simulink model "ACC_mod"  (R2025b)
settings: Solver=FixedStepAuto  StartTime=0  StopTime=SVT_StopTime  FixedStep=0.01  RelTol=1e-3
undefined symbols (not defined in the file): SVT_StepTime
settings Model: DataDictionary=ACC.sldd  Creator=spadhi  LastModifiedBy=spadhi
settings DataIOCC: TimeSaveName=SVT_tout  SignalLoggingName=SVT_logsout  DSMLoggingName=SVT_dsmout
settings DebuggingCC: SignalRangeChecking=warning  ModelReferenceIOMismatchMessage=error
settings ModelReferenceCC: UpdateModelReferenceTargets=IfOutOfDate  ModelReferenceNumInstancesAllowed=Single
settings ConfigComp: CovEnable=on  CovScope=ReferencedModels  CovIncludeTopModel=off  CovMetricSettings=dcmwe  CovHTMLOptions=-sRT=0 -sVT=0 -aTS=1 -bRG=1 -bTC=1 -hTR=0 -nFC=0 -scm=1 -bcm=1 -xEv=0  CovCumulativeReport=on  CovModelRefEnable=all

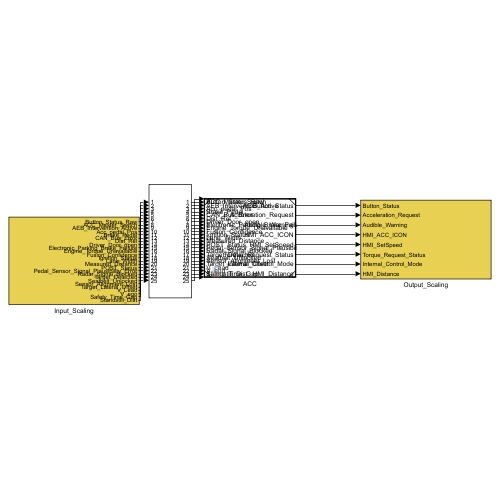
[thumbnail: Simulink's stored preview of the top-level diagram]
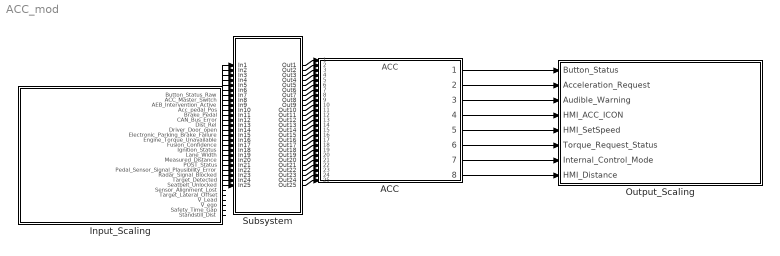
== system ACC_mod ==
  ACC : ModelReference  ModelNameDialog=ACC.slx  SimulationMode=Normal  ModelReferenceVersion=1.273
  Input_Scaling : Subsystem
  Output_Scaling : Subsystem
  Subsystem : Subsystem
  wires:
  Input_Scaling/1(Button_Status_Raw) -> Subsystem/1(In1)
  Input_Scaling/2(ACC_Master_Switch) -> Subsystem/2(In2)
  Input_Scaling/3(AEB_Intervention_Active) -> Subsystem/3(In3)
  Input_Scaling/4(Acc_pedal_Pos) -> Subsystem/4(In4)
  Input_Scaling/5(Brake_Pedal) -> Subsystem/5(In5)
  Input_Scaling/6(CAN_Bus_Error) -> Subsystem/6(In6)
  Input_Scaling/7(Dist_Rel) -> Subsystem/7(In7)
  Input_Scaling/8(Driver_Door_open) -> Subsystem/8(In8)
  Input_Scaling/9(Electronic_Parking_Brake_Failure) -> Subsystem/9(In9)
  Input_Scaling/10(Engine_Torque_Unavailable) -> Subsystem/10(In10)
  Input_Scaling/11(Fusion_Confidence) -> Subsystem/11(In11)
  Input_Scaling/12(Ignition_Status) -> Subsystem/12(In12)
  Input_Scaling/13(Lane_Width) -> Subsystem/13(In13)
  Input_Scaling/14(Measured_Distance) -> Subsystem/14(In14)
  Input_Scaling/15(POST_Status) -> Subsystem/15(In15)
  Input_Scaling/16(Pedal_Sensor_Signal_Plausibility_Error) -> Subsystem/16(In16)
  Input_Scaling/17(Radar_Signal_Blocked) -> Subsystem/17(In17)
  Input_Scaling/18(Target_Detected) -> Subsystem/18(In18)
  Input_Scaling/19(Seatbelt_Unlocked) -> Subsystem/19(In19)
  Input_Scaling/20(Sensor_Alignment_Lost) -> Subsystem/20(In20)
  Input_Scaling/21(Target_Lateral_Offset) -> Subsystem/21(In21)
  Input_Scaling/22(V_Lead) -> Subsystem/22(In22)
  Input_Scaling/23(V_ego) -> Subsystem/23(In23)
  Input_Scaling/24(Safety_Time_Gap) -> Subsystem/24(In24)
  Input_Scaling/25(Standstill_Dist) -> Subsystem/25(In25)
  Subsystem/1(Out1) -> ACC/1
  Subsystem/2(Out2) -> ACC/2
  Subsystem/3(Out3) -> ACC/3
  Subsystem/4(Out4) -> ACC/4
  Subsystem/5(Out5) -> ACC/5
  Subsystem/6(Out6) -> ACC/6
  Subsystem/7(Out7) -> ACC/7
  Subsystem/8(Out8) -> ACC/8
  Subsystem/9(Out9) -> ACC/9
  Subsystem/10(Out10) -> ACC/10
  Subsystem/11(Out11) -> ACC/11
  Subsystem/12(Out12) -> ACC/12
  Subsystem/13(Out13) -> ACC/13
  Subsystem/14(Out14) -> ACC/14
  Subsystem/15(Out15) -> ACC/15
  Subsystem/16(Out16) -> ACC/16
  Subsystem/17(Out17) -> ACC/17
  Subsystem/18(Out18) -> ACC/18
  Subsystem/19(Out19) -> ACC/19
  Subsystem/20(Out20) -> ACC/20
  Subsystem/21(Out21) -> ACC/21
  Subsystem/22(Out22) -> ACC/22
  Subsystem/23(Out23) -> ACC/23
  Subsystem/24(Out24) -> ACC/24
  Subsystem/25(Out25) -> ACC/25
  ACC/1 -> Output_Scaling/1(Button_Status)
  ACC/2 -> Output_Scaling/2(Acceleration_Request)
  ACC/3 -> Output_Scaling/3(Audible_Warning)
  ACC/4 -> Output_Scaling/4(HMI_ACC_ICON)
  ACC/5 -> Output_Scaling/5(HMI_SetSpeed)
  ACC/6 -> Output_Scaling/6(Torque_Request_Status)
  ACC/7 -> Output_Scaling/7(Internal_Control_Mode)
  ACC/8 -> Output_Scaling/8(HMI_Distance)

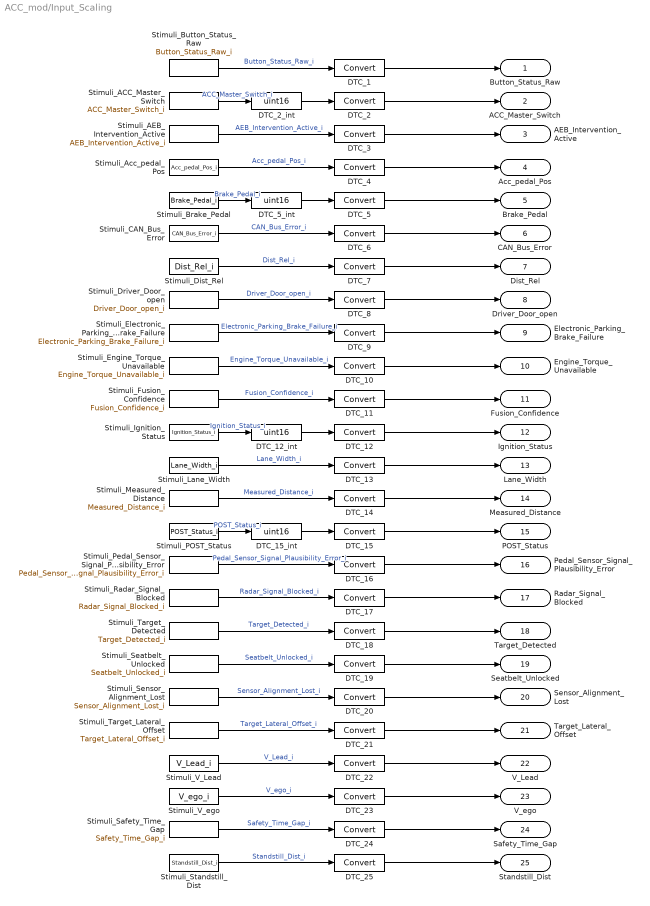
== system ACC_mod/Input_Scaling ==
  DTC_{1..25} (25 alike) : DataTypeConversion  RndMeth=Nearest  SaturateOnIntegerOverflow=off
  DTC_12_int : DataTypeConversion  OutDataTypeStr=uint16  RndMeth=Nearest  SaturateOnIntegerOverflow=off
  DTC_15_int : DataTypeConversion  OutDataTypeStr=uint16  RndMeth=Nearest  SaturateOnIntegerOverflow=off
  DTC_2_int : DataTypeConversion  OutDataTypeStr=uint16  RndMeth=Nearest  SaturateOnIntegerOverflow=off
  DTC_5_int : DataTypeConversion  OutDataTypeStr=uint16  RndMeth=Nearest  SaturateOnIntegerOverflow=off
  Stimuli_ACC_Master_Switch : FromWorkspace  VariableName=ACC_Master_Switch_i  SampleTime=SVT_StepTime  Interpolate=off  OutputAfterFinalValue=Holding final value
  Stimuli_AEB_Intervention_Active : FromWorkspace  VariableName=AEB_Intervention_Active_i  SampleTime=SVT_StepTime  Interpolate=off  OutputAfterFinalValue=Holding final value
  Stimuli_Acc_pedal_Pos : FromWorkspace  VariableName=Acc_pedal_Pos_i  SampleTime=SVT_StepTime  Interpolate=off  OutputAfterFinalValue=Holding final value
  Stimuli_Brake_Pedal : FromWorkspace  VariableName=Brake_Pedal_i  SampleTime=SVT_StepTime  Interpolate=off  OutputAfterFinalValue=Holding final value
  Stimuli_Button_Status_Raw : FromWorkspace  VariableName=Button_Status_Raw_i  SampleTime=SVT_StepTime  Interpolate=off  OutputAfterFinalValue=Holding final value
  Stimuli_CAN_Bus_Error : FromWorkspace  VariableName=CAN_Bus_Error_i  SampleTime=SVT_StepTime  Interpolate=off  OutputAfterFinalValue=Holding final value
  Stimuli_Dist_Rel : FromWorkspace  VariableName=Dist_Rel_i  SampleTime=SVT_StepTime  Interpolate=off  OutputAfterFinalValue=Holding final value
  Stimuli_Driver_Door_open : FromWorkspace  VariableName=Driver_Door_open_i  SampleTime=SVT_StepTime  Interpolate=off  OutputAfterFinalValue=Holding final value
  Stimuli_Electronic_Parking_Brake_Failure : FromWorkspace  VariableName=Electronic_Parking_Brake_Failure_i  SampleTime=SVT_StepTime  Interpolate=off  OutputAfterFinalValue=Holding final value
  Stimuli_Engine_Torque_Unavailable : FromWorkspace  VariableName=Engine_Torque_Unavailable_i  SampleTime=SVT_StepTime  Interpolate=off  OutputAfterFinalValue=Holding final value
  Stimuli_Fusion_Confidence : FromWorkspace  VariableName=Fusion_Confidence_i  SampleTime=SVT_StepTime  Interpolate=off  OutputAfterFinalValue=Holding final value
  Stimuli_Ignition_Status : FromWorkspace  VariableName=Ignition_Status_i  SampleTime=SVT_StepTime  Interpolate=off  OutputAfterFinalValue=Holding final value
  Stimuli_Lane_Width : FromWorkspace  VariableName=Lane_Width_i  SampleTime=SVT_StepTime  Interpolate=off  OutputAfterFinalValue=Holding final value
  Stimuli_Measured_Distance : FromWorkspace  VariableName=Measured_Distance_i  SampleTime=SVT_StepTime  Interpolate=off  OutputAfterFinalValue=Holding final value
  Stimuli_POST_Status : FromWorkspace  VariableName=POST_Status_i  SampleTime=SVT_StepTime  Interpolate=off  OutputAfterFinalValue=Holding final value
  Stimuli_Pedal_Sensor_Signal_Plausibility_Error : FromWorkspace  VariableName=Pedal_Sensor_Signal_Plausibility_Error_i  SampleTime=SVT_StepTime  Interpolate=off  OutputAfterFinalValue=Holding final value
  Stimuli_Radar_Signal_Blocked : FromWorkspace  VariableName=Radar_Signal_Blocked_i  SampleTime=SVT_StepTime  Interpolate=off  OutputAfterFinalValue=Holding final value
  Stimuli_Safety_Time_Gap : FromWorkspace  VariableName=Safety_Time_Gap_i  SampleTime=SVT_StepTime  Interpolate=off  OutputAfterFinalValue=Holding final value
  Stimuli_Seatbelt_Unlocked : FromWorkspace  VariableName=Seatbelt_Unlocked_i  SampleTime=SVT_StepTime  Interpolate=off  OutputAfterFinalValue=Holding final value
  Stimuli_Sensor_Alignment_Lost : FromWorkspace  VariableName=Sensor_Alignment_Lost_i  SampleTime=SVT_StepTime  Interpolate=off  OutputAfterFinalValue=Holding final value
  Stimuli_Standstill_Dist : FromWorkspace  VariableName=Standstill_Dist_i  SampleTime=SVT_StepTime  Interpolate=off  OutputAfterFinalValue=Holding final value
  Stimuli_Target_Detected : FromWorkspace  VariableName=Target_Detected_i  SampleTime=SVT_StepTime  Interpolate=off  OutputAfterFinalValue=Holding final value
  Stimuli_Target_Lateral_Offset : FromWorkspace  VariableName=Target_Lateral_Offset_i  SampleTime=SVT_StepTime  Interpolate=off  OutputAfterFinalValue=Holding final value
  Stimuli_V_Lead : FromWorkspace  VariableName=V_Lead_i  SampleTime=SVT_StepTime  Interpolate=off  OutputAfterFinalValue=Holding final value
  Stimuli_V_ego : FromWorkspace  VariableName=V_ego_i  SampleTime=SVT_StepTime  Interpolate=off  OutputAfterFinalValue=Holding final value
  Button_Status_Raw : Outport  PortDimensions=1
  ACC_Master_Switch : Outport  Port=2  PortDimensions=1
  AEB_Intervention_Active : Outport  Port=3  PortDimensions=1
  Acc_pedal_Pos : Outport  Port=4  PortDimensions=1
  Brake_Pedal : Outport  Port=5  PortDimensions=1
  CAN_Bus_Error : Outport  Port=6  PortDimensions=1
  Dist_Rel : Outport  Port=7  PortDimensions=1
  Driver_Door_open : Outport  Port=8  PortDimensions=1
  Electronic_Parking_Brake_Failure : Outport  Port=9  PortDimensions=1
  Engine_Torque_Unavailable : Outport  Port=10  PortDimensions=1
  Fusion_Confidence : Outport  Port=11  PortDimensions=1
  Ignition_Status : Outport  Port=12  PortDimensions=1
  Lane_Width : Outport  Port=13  PortDimensions=1
  Measured_Distance : Outport  Port=14  PortDimensions=1
  POST_Status : Outport  Port=15  PortDimensions=1
  Pedal_Sensor_Signal_Plausibility_Error : Outport  Port=16  PortDimensions=1
  Radar_Signal_Blocked : Outport  Port=17  PortDimensions=1
  Target_Detected : Outport  Port=18  PortDimensions=1
  Seatbelt_Unlocked : Outport  Port=19  PortDimensions=1
  Sensor_Alignment_Lost : Outport  Port=20  PortDimensions=1
  Target_Lateral_Offset : Outport  Port=21  PortDimensions=1
  V_Lead : Outport  Port=22  PortDimensions=1
  V_ego : Outport  Port=23  PortDimensions=1
  Safety_Time_Gap : Outport  Port=24  PortDimensions=1
  Standstill_Dist : Outport  Port=25  PortDimensions=1
  wires:
  Stimuli_Button_Status_Raw/1 -> DTC_1/1  "Button_Status_Raw_i"
  DTC_1/1 -> Button_Status_Raw/1
  DTC_2_int/1 -> DTC_2/1
  Stimuli_ACC_Master_Switch/1 -> DTC_2_int/1  "ACC_Master_Switch_i"
  DTC_2/1 -> ACC_Master_Switch/1
  Stimuli_AEB_Intervention_Active/1 -> DTC_3/1  "AEB_Intervention_Active_i"
  DTC_3/1 -> AEB_Intervention_Active/1
  Stimuli_Acc_pedal_Pos/1 -> DTC_4/1  "Acc_pedal_Pos_i"
  DTC_4/1 -> Acc_pedal_Pos/1
  DTC_5_int/1 -> DTC_5/1
  Stimuli_Brake_Pedal/1 -> DTC_5_int/1  "Brake_Pedal_i"
  DTC_5/1 -> Brake_Pedal/1
  Stimuli_CAN_Bus_Error/1 -> DTC_6/1  "CAN_Bus_Error_i"
  DTC_6/1 -> CAN_Bus_Error/1
  Stimuli_Dist_Rel/1 -> DTC_7/1  "Dist_Rel_i"
  DTC_7/1 -> Dist_Rel/1
  Stimuli_Driver_Door_open/1 -> DTC_8/1  "Driver_Door_open_i"
  DTC_8/1 -> Driver_Door_open/1
  Stimuli_Electronic_Parking_Brake_Failure/1 -> DTC_9/1  "Electronic_Parking_Brake_Failure_i"
  DTC_9/1 -> Electronic_Parking_Brake_Failure/1
  Stimuli_Engine_Torque_Unavailable/1 -> DTC_10/1  "Engine_Torque_Unavailable_i"
  DTC_10/1 -> Engine_Torque_Unavailable/1
  Stimuli_Fusion_Confidence/1 -> DTC_11/1  "Fusion_Confidence_i"
  DTC_11/1 -> Fusion_Confidence/1
  DTC_12_int/1 -> DTC_12/1
  Stimuli_Ignition_Status/1 -> DTC_12_int/1  "Ignition_Status_i"
  DTC_12/1 -> Ignition_Status/1
  Stimuli_Lane_Width/1 -> DTC_13/1  "Lane_Width_i"
  DTC_13/1 -> Lane_Width/1
  Stimuli_Measured_Distance/1 -> DTC_14/1  "Measured_Distance_i"
  DTC_14/1 -> Measured_Distance/1
  DTC_15_int/1 -> DTC_15/1
  Stimuli_POST_Status/1 -> DTC_15_int/1  "POST_Status_i"
  DTC_15/1 -> POST_Status/1
  Stimuli_Pedal_Sensor_Signal_Plausibility_Error/1 -> DTC_16/1  "Pedal_Sensor_Signal_Plausibility_Error_i"
  DTC_16/1 -> Pedal_Sensor_Signal_Plausibility_Error/1
  Stimuli_Radar_Signal_Blocked/1 -> DTC_17/1  "Radar_Signal_Blocked_i"
  DTC_17/1 -> Radar_Signal_Blocked/1
  Stimuli_Target_Detected/1 -> DTC_18/1  "Target_Detected_i"
  DTC_18/1 -> Target_Detected/1
  Stimuli_Seatbelt_Unlocked/1 -> DTC_19/1  "Seatbelt_Unlocked_i"
  DTC_19/1 -> Seatbelt_Unlocked/1
  Stimuli_Sensor_Alignment_Lost/1 -> DTC_20/1  "Sensor_Alignment_Lost_i"
  DTC_20/1 -> Sensor_Alignment_Lost/1
  Stimuli_Target_Lateral_Offset/1 -> DTC_21/1  "Target_Lateral_Offset_i"
  DTC_21/1 -> Target_Lateral_Offset/1
  Stimuli_V_Lead/1 -> DTC_22/1  "V_Lead_i"
  DTC_22/1 -> V_Lead/1
  Stimuli_V_ego/1 -> DTC_23/1  "V_ego_i"
  DTC_23/1 -> V_ego/1
  Stimuli_Safety_Time_Gap/1 -> DTC_24/1  "Safety_Time_Gap_i"
  DTC_24/1 -> Safety_Time_Gap/1
  Stimuli_Standstill_Dist/1 -> DTC_25/1  "Standstill_Dist_i"
  DTC_25/1 -> Standstill_Dist/1

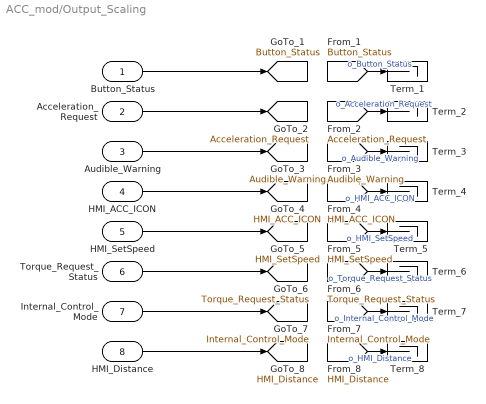
== system ACC_mod/Output_Scaling ==
  Button_Status : Inport
  Acceleration_Request : Inport  Port=2
  Audible_Warning : Inport  Port=3
  HMI_ACC_ICON : Inport  Port=4
  HMI_SetSpeed : Inport  Port=5
  Torque_Request_Status : Inport  Port=6
  Internal_Control_Mode : Inport  Port=7
  HMI_Distance : Inport  Port=8
  Term_{1..8} (8 alike) : Terminator
  tag scope: Acceleration_Request=global, Audible_Warning=global, Button_Status=global, HMI_ACC_ICON=global, HMI_Distance=global, HMI_SetSpeed=global, Internal_Control_Mode=global, Torque_Request_Status=global
  wires:
  Button_Status/1 -> [Button_Status]
  [Button_Status] -> Term_1/1  "o_Button_Status"
  Acceleration_Request/1 -> [Acceleration_Request]
  [Acceleration_Request] -> Term_2/1  "o_Acceleration_Request"
  Audible_Warning/1 -> [Audible_Warning]
  [Audible_Warning] -> Term_3/1  "o_Audible_Warning"
  HMI_ACC_ICON/1 -> [HMI_ACC_ICON]
  [HMI_ACC_ICON] -> Term_4/1  "o_HMI_ACC_ICON"
  HMI_SetSpeed/1 -> [HMI_SetSpeed]
  [HMI_SetSpeed] -> Term_5/1  "o_HMI_SetSpeed"
  Torque_Request_Status/1 -> [Torque_Request_Status]
  [Torque_Request_Status] -> Term_6/1  "o_Torque_Request_Status"
  Internal_Control_Mode/1 -> [Internal_Control_Mode]
  [Internal_Control_Mode] -> Term_7/1  "o_Internal_Control_Mode"
  HMI_Distance/1 -> [HMI_Distance]
  [HMI_Distance] -> Term_8/1  "o_HMI_Distance"

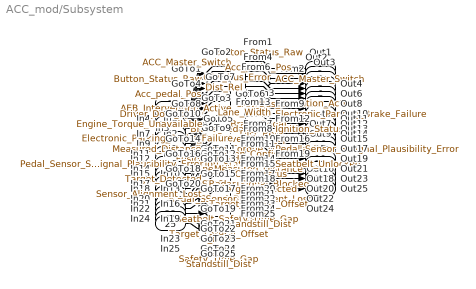
== system ACC_mod/Subsystem ==
  In1 : Inport
  In2 : Inport  Port=2
  In3 : Inport  Port=3
  In4 : Inport  Port=4
  In5 : Inport  Port=5
  In6 : Inport  Port=6
  In7 : Inport  Port=7
  In8 : Inport  Port=8
  In9 : Inport  Port=9
  In10 : Inport  Port=10
  In11 : Inport  Port=11
  In12 : Inport  Port=12
  In13 : Inport  Port=13
  In14 : Inport  Port=14
  In15 : Inport  Port=15
  In16 : Inport  Port=16
  In17 : Inport  Port=17
  In18 : Inport  Port=18
  In19 : Inport  Port=19
  In20 : Inport  Port=20
  In21 : Inport  Port=21
  In22 : Inport  Port=22
  In23 : Inport  Port=23
  In24 : Inport  Port=24
  In25 : Inport  Port=25
  Out1 : Outport
  Out2 : Outport  Port=2
  Out3 : Outport  Port=3
  Out4 : Outport  Port=4
  Out5 : Outport  Port=5
  Out6 : Outport  Port=6
  Out7 : Outport  Port=7
  Out8 : Outport  Port=8
  Out9 : Outport  Port=9
  Out10 : Outport  Port=10
  Out11 : Outport  Port=11
  Out12 : Outport  Port=12
  Out13 : Outport  Port=13
  Out14 : Outport  Port=14
  Out15 : Outport  Port=15
  Out16 : Outport  Port=16
  Out17 : Outport  Port=17
  Out18 : Outport  Port=18
  Out19 : Outport  Port=19
  Out20 : Outport  Port=20
  Out21 : Outport  Port=21
  Out22 : Outport  Port=22
  Out23 : Outport  Port=23
  Out24 : Outport  Port=24
  Out25 : Outport  Port=25
  tag scope: ACC_Master_Switch=global, AEB_Intervention_Active=global, Acc_pedal_Pos=global, Brake_Pedal=global, Button_Status_Raw=global, CAN_Bus_Error=global, Dist_Rel=global, Driver_Door_open=global, Electronic_Parking_Brake_Failure=global, Engine_Torque_Unavailable=global, Fusion_Confidence=global, Ignition_Status=global, Lane_Width=global, Measured_Distance=global, POST_Status=global, Pedal_Sensor_Signal_Plausibility_Error=global, Radar_Signal_Blocked=global, Safety_Time_Gap=global, Seatbelt_Unlocked=global, Sensor_Alignment_Lost=global, Standstill_Dist=global, Target_Detected=global, Target_Lateral_Offset=global, V_Lead=global, V_ego=global
  wires:
  In4/1 -> [Acc_pedal_Pos]
  In23/1 -> [V_ego]
  In7/1 -> [Dist_Rel]
  In5/1 -> [Brake_Pedal]
  [Target_Detected] -> Out18/1
  In2/1 -> [ACC_Master_Switch]
  In9/1 -> [Electronic_Parking_Brake_Failure]
  In12/1 -> [Ignition_Status]
  In24/1 -> [Safety_Time_Gap]
  In22/1 -> [V_Lead]
  In16/1 -> [Pedal_Sensor_Signal_Plausibility_Error]
  In6/1 -> [CAN_Bus_Error]
  [Sensor_Alignment_Lost] -> Out20/1
  [Pedal_Sensor_Signal_Plausibility_Error] -> Out16/1
  [Brake_Pedal] -> Out5/1
  [Ignition_Status] -> Out12/1
  [Dist_Rel] -> Out7/1
  In20/1 -> [Sensor_Alignment_Lost]
  In11/1 -> [Fusion_Confidence]
  In25/1 -> [Standstill_Dist]
  [Fusion_Confidence] -> Out11/1
  [Acc_pedal_Pos] -> Out4/1
  In15/1 -> [POST_Status]
  In10/1 -> [Engine_Torque_Unavailable]
  In21/1 -> [Target_Lateral_Offset]
  In3/1 -> [AEB_Intervention_Active]
  In18/1 -> [Target_Detected]
  In19/1 -> [Seatbelt_Unlocked]
  [Standstill_Dist] -> Out25/1
  [Engine_Torque_Unavailable] -> Out10/1
  In1/1 -> [Button_Status_Raw]
  In14/1 -> [Measured_Distance]
  [Measured_Distance] -> Out14/1
  [Seatbelt_Unlocked] -> Out19/1
  In13/1 -> [Lane_Width]
  [ACC_Master_Switch] -> Out2/1
  [CAN_Bus_Error] -> Out6/1
  [POST_Status] -> Out15/1
  In8/1 -> [Driver_Door_open]
  [Radar_Signal_Blocked] -> Out17/1
  [Driver_Door_open] -> Out8/1
  [Electronic_Parking_Brake_Failure] -> Out9/1
  In17/1 -> [Radar_Signal_Blocked]
  [AEB_Intervention_Active] -> Out3/1
  [Safety_Time_Gap] -> Out24/1
  [Lane_Width] -> Out13/1
  [V_ego] -> Out23/1
  [V_Lead] -> Out22/1
  [Button_Status_Raw] -> Out1/1
  [Target_Lateral_Offset] -> Out21/1
